simulink model "Design_5new_4weeks_Q3"  (R2026a)
settings: Solver=FixedStepAuto  StopTime=2419200  FixedStep=300
undefined symbols (not defined in the file): coloring, m, n, tamk, vapor
libraries: mqttlib x7
(part 1 of 2)
settings Model: Creator=User  LastModifiedBy=User
settings ConfigComp: PLC_TargetIDE=codesys35  PLC_MultiTBSigbuilderTimeRange=off  PLC_FoldFBCallOutputVar=off  PLC_RemoveUnusedSSMethodCallArguments=off  PLC_UseCallOutputArgSyntax=off  PLC_EnableUnsignedAndDoubleTypes=off  PLC_EnableUDTSplitting=off  PLC_MaxFieldsInUDT=500.0  PLC_InlineEnumCastFunction=off  PLC_RTWMaxIdLength=31.0  PLC_RollThreshold=5.0  PLC_ActiveTab=0.0  PLC_EnableStringLiteralTB=on  PLC_Enable64bitIntSupport=off

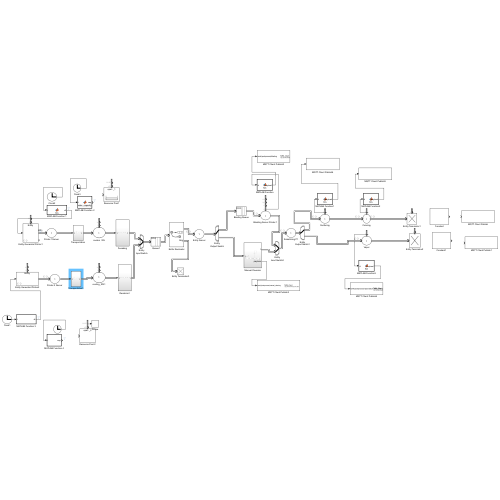
[thumbnail: Simulink's stored preview of the top-level diagram]
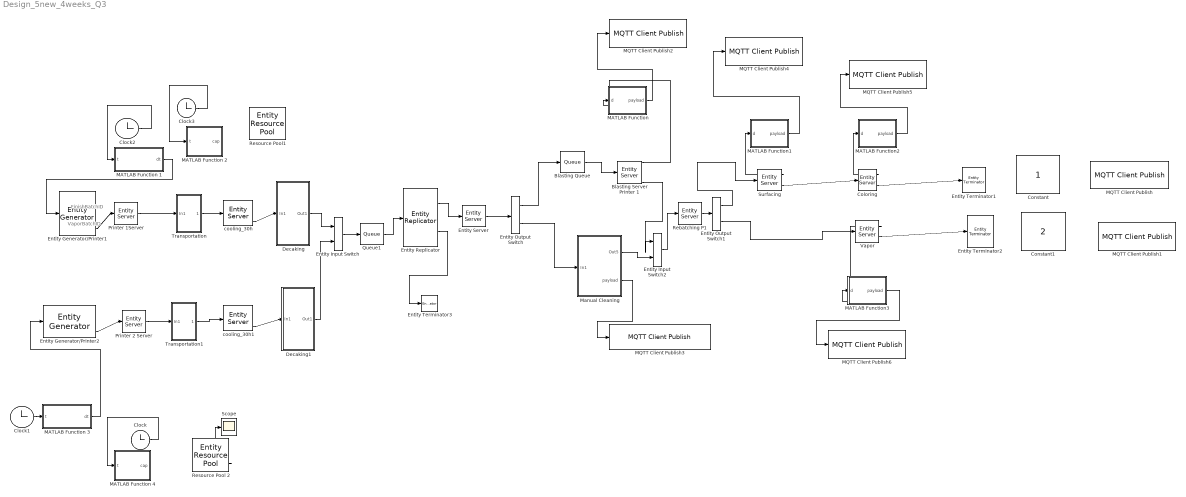
== system Design_5new_4weeks_Q3 ==
  note: VaporBatchID
  note: FinishBatchID
  " Queue1" : Queue  InputPortMessageModes=m  OutputPortMessageModes=m
  Blasting Queue : Queue  InputPortMessageModes=m  OutputPortMessageModes=m
  Blasting Server Printer 1 : EntityServer  InputPortMessageModes=m  OutputPortMessageModes=n,n,n,n,m  Capacity=1  ServiceTimeValue=8*60  EntryAction=|  NumberEntitiesDeparted=on  NumberEntitiesInBlock=on  NumberEntitiesPending=on  NumEntitiesExtracted=on
      | % =========================================================
      | % BLASTING PROCESS : PowerShot C
      | % Supervisor Excel Values
      | % Simulink-safe version
      | % =========================================================
      | 
      | entity.prev_proc = 3;          % 3 = Blasting completed
      | 
      | % Supervisor values
      | entity.operator_time_min = 1;  % min/batch
      | entity.capacity_L = 5;         % L/batch
      | entity.process_time_min = 8;   % min
      | entity.power = 5;              % kW
      | 
      | % Energy calculation
      | entity.energy = ...
      |     entity.power * entity.process_time_min / 60;
      | 
      | % Accumulate totals
      | entity.total_energy = ...
      |     entity.total_energy + entity.energy;
      | 
      | entity.total_operator_min = ...
      |     entity.total_operator_min + entity.operator_time_min;
      | 
      | % Debug print
      | fprintf(['[BLASTING CHECK] ' ...
      |     'SourceID=%g | BuildID=%g | BatchID=%g | PartID=%g | ' ...
      |     'PrevProc=%g | Volume=%.2f | Capacity=%.2f | ' ...
      |     'ProcessTime=%.2f min | Operator=%.2f min | ' ...
      |     'Power=%.2f kW | Energy=%.3f kWh | ' ...
      |     'TotalEnergy=%.3f kWh | TotalOperator=%.3f min\n'], ...
      |     entity.SourceID, ...
      |     entity.BuildID, ...
      |     entity.BatchID, ...
      |     entity.PartID, ...
      |     entity.prev_proc, ...
      |     entity.part_volume, ...
      |     entity.capacity_L, ...
      |     entity.process_time_min, ...
      |     entity.operator_time_min, ...
      |     entity.power, ...
      |     entity.energy, ...
      |     entity.total_energy, ...
      |     entity.total_operator_min);
      settings: OutputPortMap=o0,o1,o3,o12,o9
  Clock{,1..3} (4 alike) : Clock
  Coloring : EntityServer  InputPortMessageModes=m  OutputPortMessageModes=n,m  Capacity=1  ServiceTimeValue=150*60  EntryAction=|  ExitAction=|  NumberEntitiesDeparted=on
      EntryAction=|
      | %#codegen
      | 
      | % =========================================================
      | % SURFACING PROCESS : PowerShot S
      | % Supervisor Excel Values
      | % Simulink-safe version
      | % =========================================================
      | 
      | persistent surfacingBatchCounter
      | 
      | if isempty(surfacingBatchCounter)
      |     surfacingBatchCounter = 9000;    % first SurfacingBatchID = 9001
      | end
      | 
      | % =========================================================
      | % DUPLICATE PROTECTION
      | % If this entity already completed Surfacing, do not add energy again
      | % =========================================================
      | if entity.prev_proc == 5
      | 
      |     fprintf(['[SURFACING SKIPPED - ALREADY DONE] ' ...
      |         'SourceID=%g | BuildID=%g | PartID=%g | BatchID=%g | TotalEnergy=%.3f\n'], ...
      |         entity.SourceID, ...
      |         entity.BuildID, ...
      |         entity.PartID, ...
      |         entity.BatchID, ...
      |         entity.total_energy);
      | 
      | else
      | 
      |     % =====================================================
      |     % PROCESS IDENTIFICATION
      |     % =====================================================
      |     entity.prev_proc = 5;          % 5 = Surfacing completed
      |     entity.process_name = 5;
      | 
      |     % =====================================================
      |     % SUPERVISOR VALUES
      |     % =====================================================
      |     entity.operator_time_min = 1;  % min/batch
      |     entity.capacity_L = 5;         % L/batch
      |     entity.process_time_min = 10;  % min
      |     entity.power = 5;              % kW
      | 
      |     % =====================================================
      |     % ENERGY CALCULATION
      |     % =====================================================
      |     entity.energy = entity.power * entity.process_time_min / 60;
      | 
      |     % =====================================================
      |     % ACCUMULATE TOTALS
      |     % =====================================================
      |     entity.total_energy = entity.total_energy + entity.energy;
      | 
      |     entity.total_operator_min = ...
      |         entity.total_operator_min + entity.operator_time_min;
      | 
      |     % =====================================================
      |     % NEW BATCH ID AFTER SURFACING
      |     % Coloring receives this BatchID
      |     % =====================================================
      |     surfacingBatchCounter = surfacingBatchCounter + 1;
      | 
      |     entity.surfacing_batch_id = surfacingBatchCounter;
      |     entity.SurfaceBatchID = surfacingBatchCounter;
      | 
      |     % Current active BatchID after Surfacing
      |     entity.BatchID = entity.surfacing_batch_id;
      | 
      |     % Keep route marker for Coloring path
      |     entity.finish_type = 1;
      | 
      |     % =====================================================
      |     % DEBUG PRINT
      |     % =====================================================
      |     fprintf(['[SURFACING CHECK] ' ...
      |         'SourceID=%g | BuildID=%g | BatchID=%g | ' ...
      |         'SurfacingBatchID=%g | ColoringInputBatchID=%g | ' ...
      |         'PartID=%g | PrevProc=%g | FinishType=%g | Volume=%.2f | Capacity=%.2f | ' ...
      |         'ProcessTime=%.2f min | Operator=%.2f min | ' ...
      |         'Power=%.2f kW | Energy=%.3f kWh | ' ...
      |         'TotalEnergy=%.3f kWh | TotalOperator=%.3f min\n'], ...
      |         entity.SourceID, ...
      |         entity.BuildID, ...
      |         entity.BatchID, ...
      |         entity.surfacing_batch_id, ...
      |         entity.BatchID, ...
      |         entity.PartID, ...
      |         entity.prev_proc, ...
      |         entity.finish_type, ...
      |         entity.part_volume, ...
      |         entity.capacity_L, ...
      |         entity.process_time_min, ...
      |         entity.operator_time_min, ...
      |         entity.power, ...
      |         entity.energy, ...
      |         entity.total_energy, ...
      |         entity.total_operator_min);
      | 
      | end
      ExitAction=|
      | fprintf('[COLORING CHECK] PartID=%g | BatchID=%g\n', ...
      |     entity.PartID, ...
      |     entity.BatchID);
      settings: OutputPortMap=o0,o9
  Constant : Constant  SampleTime=300
  Constant1 : Constant  Value=2  SampleTime=300
  Decaking : Subsystem
  Decaking1 : Subsystem
  Entity Input Switch : EntityInputSwitch  InputPortMessageModes=m,m  OutputPortMessageModes=m
  Entity Input Switch2 : EntityInputSwitch  InputPortMessageModes=m,m  OutputPortMessageModes=m
  Entity Output Switch : EntityOutputSwitch  InputPortMessageModes=m  OutputPortMessageModes=m,m  SwitchingCriterion=From attribute  SwitchAttributeName=route_dp
  Entity Output Switch1 : EntityOutputSwitch  InputPortMessageModes=m  OutputPortMessageModes=m,m  SwitchingCriterion=From attribute  SwitchAttributeName=finish_type
  Entity Generator/Printer1 : EntityGenerator  OutputPortMessageModes=n,n,m  TimeSource=Signal port  GenerateAction=|  AttributeName=BatchID|PartID|material_type|finish_type|prev_proc|SourceID|route_dp|BuildID|part_volume|blast_batch_id|manual_batch_id|surface_batch_id|vapor_batch_id|Build_Time|Build_Volume|Build_schedule|Primary_powder|Secondary_powder|Inert_gas_cons|Electricity_cons|Comp_air_cons|Fill_ratio|Build_height|Laser_power|Total_print_mass|Heat_loss|process_time_min|operator_time_min|capacity_L|power|energy|transport_time_min|total_energy|total_operator_min|process_name|energy_stage|finish_batch_id|PrinterBatchID|DecakingBatchID|RouteID|FinishBatchI|ColorBatchID|FinalBatchID|BlastBatchID|ManualBatchID|FinishBatchID|SurfaceBatchID|VaporBatchID|printer_batch_id|color_batch_id|surfacing_batch_id  AttributeInitialValue=0|0|1|2|1|0|1|0|0|0|0|0|0|0|0|1|0|0|0|0|0|0|0|0|0|0|0|0|0|0|0|10|0|0|0|0|0|0|0|0|0|0|0|0|0|0|0|0|0|0|0  NumberEntitiesDeparted=on  AverageIntergenerationTime=on  EntityType=Structured  EntityTypeName=Entity
      | %#codegen
      | 
      | persistent batchCounter1 printer1PrintDone
      | 
      | % =========================================================
      | % INIT
      | % =========================================================
      | if isempty(batchCounter1)
      |     batchCounter1 = 0;
      | end
      | 
      | if isempty(printer1PrintDone)
      |     printer1PrintDone = false;
      | end
      | 
      | batchCounter1 = batchCounter1 + 1;
      | 
      | % =========================================================
      | % BASIC IDs
      | % =========================================================
      | entity.SourceID = 1;
      | entity.PartID   = 0;
      | 
      | entity.BuildID = batchCounter1;
      | entity.BatchID = 0;
      | 
      | % =========================================================
      | % INITIALIZE ALL BATCH FIELDS
      | % =========================================================
      | entity.PrinterBatchID  = batchCounter1;
      | entity.DecakingBatchID = 0;
      | entity.RouteID         = 0;
      | 
      | entity.BlastBatchID    = 0;
      | entity.ManualBatchID   = 0;
      | entity.FinishBatchID   = 0;
      | entity.SurfaceBatchID  = 0;
      | entity.VaporBatchID    = 0;
      | entity.ColorBatchID    = 0;
      | entity.FinalBatchID    = 0;
      | 
      | % lowercase fields, if used in later blocks
      | entity.printer_batch_id   = batchCounter1;
      | entity.color_batch_id     = 0;
      | entity.surfacing_batch_id = 0;
      | 
      | % =========================================================
      | % BUILD / PRINTER
      | % =========================================================
      | entity.Build_Time     = 1200;      % min = 20 h
      | entity.Build_Volume   = 10000;     % cm3
      | entity.Build_schedule = 1;
      | 
      | % =========================================================
      | % PART
      | % =========================================================
      | entity.part_volume   = 0;
      | entity.material_type = 1;
      | 
      | % =========================================================
      | % ROUTING DEFAULTS
      | % =========================================================
      | entity.prev_proc   = 1;    % 1 = Printing completed
      | entity.route_dp    = 1;
      | entity.finish_type = 1;
      | 
      | % =========================================================
      | % PROCESS PARAMETERS
      | % =========================================================
      | entity.power            = 2;       % kW
      | entity.process_time_min = 1200;    % min
      | 
      | % =========================================================
      | % ENERGY
      | % =========================================================
      | entity.energy = entity.power * entity.process_time_min / 60;
      | entity.total_energy = entity.energy;
      | 
      | % =========================================================
      | % OPERATOR / TRANSPORT
      | % =========================================================
      | entity.operator_time_min  = 0;
      | entity.capacity_L         = 0;
      | entity.transport_time_min = 10;
      | entity.total_operator_min = 0;
      | 
      | % =========================================================
      | % DEBUG / TRACKING
      | % =========================================================
      | entity.energy_stage = 1;
      | entity.process_name = 1;
      | 
      | % =========================================================
      | % DEBUG PRINT ONLY ONCE
      | % =========================================================
      | if ~printer1PrintDone
      |     fprintf('[Printer1 INIT] SourceID=%g | BuildID=%g | BatchID=%g | PrinterBatchID=%g | PartID=%g | BuildTime=%g min | Energy=%.3f | Total=%.3f\n', ...
      |         entity.SourceID, ...
      |         entity.BuildID, ...
      |         entity.BatchID, ...
      |         entity.PrinterBatchID, ...
      |         entity.PartID, ...
      |         entity.process_time_min, ...
      |         entity.energy, ...
      |         entity.total_energy);
      | 
      |     printer1PrintDone = true;
      | end
      settings: InputPortMap=u1  OutputPortMap=o0,o2,o3
  Entity Generator/Printer2 : EntityGenerator  OutputPortMessageModes=n,n,m  TimeSource=Signal port  GenerateAction=|  AttributeName=BatchID|PartID|material_type|finish_type|prev_proc|SourceID|route_dp|BuildID|part_volume|blast_batch_id|manual_batch_id|surface_batch_id|vapor_batch_id|Build_Time|Build_Volume|Build_schedule|Primary_powder|Secondary_powder|Inert_gas_cons|Electricity_cons|Comp_air_cons|Fill_ratio|Build_height|Laser_power|Total_print_mass|Heat_loss|process_time_min|operator_time_min|capacity_L|power|energy|transport_time_min|total_energy|total_operator_min|process_name|energy_stage|finish_batch_id|PrinterBatchID|DecakingBatchID|RouteID|FinishBatchI|ColorBatchID|FinalBatchID|BlastBatchID|ManualBatchID|FinishBatchID|SurfaceBatchID|VaporBatchID|printer_batch_id|color_batch_id|surfacing_batch_id  AttributeInitialValue=0|1|0|2|1|0|1|0|0|0|0|0|0|0|0|1|0|0|0|0|0|0|0|0|0|0|0|0|0|0|0|10|0|0|0|0|0|0|0|0|0|0|0|0|0|0|0|0|0|0|0  NumberEntitiesDeparted=on  AverageIntergenerationTime=on  EntityType=Structured  EntityTypeName=Entity
      | %#codegen
      | 
      | persistent batchCounter2 printer2PrintDone
      | 
      | % =========================================================
      | % INIT
      | % =========================================================
      | if isempty(batchCounter2)
      |     batchCounter2 = 999;      % first BuildID = 1000
      | end
      | 
      | if isempty(printer2PrintDone)
      |     printer2PrintDone = false;
      | end
      | 
      | batchCounter2 = batchCounter2 + 1;
      | 
      | % =========================================================
      | % BASIC IDs
      | % =========================================================
      | entity.SourceID = 2;
      | entity.PartID   = 0;
      | 
      | % Build tracking
      | entity.BuildID = batchCounter2;
      | 
      | % Current/latest batch ID
      | entity.BatchID = 0;
      | 
      | % =========================================================
      | % INITIALIZE ALL BATCH FIELDS
      | % =========================================================
      | entity.PrinterBatchID  = batchCounter2;
      | entity.DecakingBatchID = 0;
      | entity.RouteID         = 0;
      | 
      | entity.BlastBatchID    = 0;
      | entity.ManualBatchID   = 0;
      | 
      | entity.FinishBatchID   = 0;
      | entity.SurfaceBatchID  = 0;
      | entity.VaporBatchID    = 0;
      | 
      | entity.ColorBatchID    = 0;
      | entity.FinalBatchID    = 0;
      | 
      | % lowercase versions used later in model
      | entity.printer_batch_id   = batchCounter2;
      | entity.color_batch_id     = 0;
      | entity.surfacing_batch_id = 0;
      | 
      | % =========================================================
      | % PRINTER / BUILD
      | % =========================================================
      | entity.Build_Time     = 1440;      % min = 24 h
      | entity.Build_Volume   = 10000;     % cm3
      | entity.Build_schedule = 1;
      | 
      | % =========================================================
      | % PART - ASSIGNED LATER
      | % =========================================================
      | entity.part_volume   = 0;
      | entity.material_type = 1;
      | 
      | % =========================================================
      | % MATERIAL / CONSUMPTION - INITIAL VALUES
      | % =========================================================
      | entity.Primary_powder   = 0;
      | entity.Secondary_powder = 0;
      | 
      | entity.Inert_gas_cons   = 0;
      | entity.Electricity_cons = 0;
      | entity.Comp_air_cons    = 0;
      | 
      | entity.Fill_ratio       = 0;
      | entity.Build_height     = 0;
      | 
      | entity.Laser_power      = 0;
      | entity.Total_print_mass = 0;
      | entity.Heat_loss        = 0;
      | 
      | % =========================================================
      | % ROUTING DEFAULT VALUES
      | % =========================================================
      | entity.prev_proc   = 1;      % 1 = Printing completed
      | entity.route_dp    = 1;
      | entity.finish_type = 1;
      | 
      | % =========================================================
      | % ENERGY
      | % =========================================================
      | entity.power = 2;                 % kW
      | 
      | entity.process_time_min = 1440;   % min
      | 
      | % Printer energy calculation
      | entity.energy = ...
      |     entity.power * entity.process_time_min / 60;
      | 
      | % Initialize total energy
      | entity.total_energy = entity.energy;
      | 
      | % =========================================================
      | % OTHER PROCESS ATTRIBUTES
      | % =========================================================
      | entity.operator_time_min  = 0;
      | 
      | entity.capacity_L         = 0;
      | 
      | entity.transport_time_min = 10;
      | 
      | entity.total_operator_min = 0;
      | 
      | % =========================================================
      | % DEBUG / TRACKING
      | % =========================================================
      | entity.energy_stage = 1;
      | 
      | entity.process_name = 1;
      | 
      | % =========================================================
      | % DEBUG PRINT ONLY ONE TIME
      | % =========================================================
      | if ~printer2PrintDone
      | 
      |     fprintf('[Printer2 INIT] SourceID=%g | BuildID=%g | BatchID=%g | PrinterBatchID=%g | PartID=%g | BuildTime=%g min | Energy=%.3f | Total=%.3f\n', ...
      |         entity.SourceID, ...
      |         entity.BuildID, ...
      |         entity.BatchID, ...
      |         entity.PrinterBatchID, ...
      |         entity.PartID, ...
      |         entity.process_time_min, ...
      |         entity.energy, ...
      |         entity.total_energy);
      | 
      |     printer2PrintDone = true;
      | 
      | end
      settings: InputPortMap=u1  OutputPortMap=o0,o2,o3
  Entity Replicator : EntityReplicator  InputPortMessageModes=m  OutputPortMessageModes=m,m  ReplicasDepartFrom=Single output port  NumberReplicas=5  HoldOriginalEntityUntilAllReplicasDepart=on
  Entity Server : EntityServer  InputPortMessageModes=m  OutputPortMessageModes=m  Capacity=1  EntryAction=|
      | persistent partCounterP1 partCounterP2
      | persistent blastBatchCounter manualBatchCounter
      | 
      | % =========================================================
      | % INIT
      | % =========================================================
      | if isempty(partCounterP1)
      |     partCounterP1 = 0;
      | end
      | 
      | if isempty(partCounterP2)
      |     partCounterP2 = 0;
      | end
      | 
      | % =========================================================
      | % NEW BATCH COUNTERS
      | % =========================================================
      | if isempty(blastBatchCounter)
      |     blastBatchCounter = 3000;
      | end
      | 
      | if isempty(manualBatchCounter)
      |     manualBatchCounter = 4000;
      | end
      | 
      | % =========================================================
      | % PART ASSIGNMENT AFTER REPLICATOR / MERGED LINE
      | % =========================================================
      | if entity.SourceID == 1
      | 
      |     partCounterP1 = partCounterP1 + 1;
      |     localIndex = mod(partCounterP1 - 1, 5) + 1;
      | 
      |     entity.PartID = localIndex;
      |     volume_map = [5 6 7 8 9];
      | 
      |     % Original printer batch
      |     entity.printer_batch_id = localIndex;
      | 
      | else
      | 
      |     partCounterP2 = partCounterP2 + 1;
      |     localIndex = mod(partCounterP2 - 1, 5) + 1;
      | 
      |     entity.PartID = localIndex + 5;
      |     volume_map = [10 11 12 13 14];
      | 
      |     % Original printer batch
      |     entity.printer_batch_id = 1000 + localIndex;
      | 
      | end
      | 
      | % =========================================================
      | % PART VOLUME
      | % =========================================================
      | entity.part_volume = volume_map(localIndex);
      | 
      | % =========================================================
      | % ROUTING LOGIC
      | % =========================================================
      | if localIndex <= 4
      | 
      |     % ============================================
      |     % BLASTING ROUTE
      |     % ============================================
      |     entity.route_dp = 1;
      |     entity.prev_proc = 1;
      | 
      |     % NEW blasting batch
      |     blastBatchCounter = blastBatchCounter + 1;
      | 
      |     entity.blast_batch_id = blastBatchCounter;
      |     entity.manual_batch_id = 0;
      | 
      |     % CURRENT ACTIVE BATCH
      |     entity.BatchID = entity.blast_batch_id;
      | 
      |     entity.process_name = 1;
      | 
      | else
      | 
      |     % ============================================
      |     % MANUAL CLEANING ROUTE
      |     % ============================================
      |     entity.route_dp = 2;
      |     entity.prev_proc = 2;
      | 
      |     % NEW manual cleaning batch
      |     manualBatchCounter = manualBatchCounter + 1;
      | 
      |     entity.manual_batch_id = manualBatchCounter;
      |     entity.blast_batch_id = 0;
      | 
      |     % CURRENT ACTIVE BATCH
      |     entity.BatchID = entity.manual_batch_id;
      | 
      |     entity.process_name = 2;
      | 
      | end
      | 
      | % =========================================================
      | % DEBUG PRINT
      | % =========================================================
      | fprintf(['[ASSIGN COMMON] SourceID=%g | BuildID=%g | ' ...
      |     'PrinterBatchID=%g | BatchID=%g | BlastBatchID=%g | ' ...
      |     'ManualBatchID=%g | PartID=%g | Volume=%.2f | ' ...
      |     'route_dp=%g | prev_proc=%g | process_name=%g | ' ...
      |     'total_energy=%.3f\n'], ...
      |     entity.SourceID, ...
      |     entity.BuildID, ...
      |     entity.printer_batch_id, ...
      |     entity.BatchID, ...
      |     entity.blast_batch_id, ...
      |     entity.manual_batch_id, ...
      |     entity.PartID, ...
      |     entity.part_volume, ...
      |     entity.route_dp, ...
      |     entity.prev_proc, ...
      |     entity.process_name, ...
      |     entity.total_energy);
  Entity Terminator1 : EntityTerminator  InputPortMessageModes=m  NumberEntitiesArrived=on
      settings: OutputPortMap=o0
  Entity Terminator2 : EntityTerminator  InputPortMessageModes=m  NumberEntitiesArrived=on
      settings: OutputPortMap=o0
  Entity Terminator3 : EntityTerminator  InputPortMessageModes=m
  MATLAB Function : MATLAB Function  TreatAsAtomicUnit=on
  MATLAB Function 1 : MATLAB Function  TreatAsAtomicUnit=on
  MATLAB Function 2 : MATLAB Function  TreatAsAtomicUnit=on
  MATLAB Function 3 : MATLAB Function  TreatAsAtomicUnit=on
  MATLAB Function 4 : MATLAB Function  TreatAsAtomicUnit=on
  MATLAB Function1 : MATLAB Function  TreatAsAtomicUnit=on
  MATLAB Function2 : MATLAB Function  TreatAsAtomicUnit=on
  MATLAB Function3 : MATLAB Function  TreatAsAtomicUnit=on
  MQTT Client Publish : mqttlib/MQTT Client Publish  RetainClient=TAMK_Client  ClientList=TAMK_Client  TopicsTable={ '1', 'tamk/coloring', '0', 'off' }  PublishOnDataChange=off  SampleTime=-1  TopicNames=tamk/coloring  NumTopics=1  IsLib=0  BlkName=MQTT Client Publish
  MQTT Client Publish1 : mqttlib/MQTT Client Publish  RetainClient=TAMK_Client  ClientList=TAMK_Client  TopicsTable={ '1', 'tamk/vapor', '0', 'off' }  PublishOnDataChange=off  SampleTime=-1  TopicNames=tamk/vapor  NumTopics=1  IsLib=0  BlkName=MQTT Client Publish
  MQTT Client Publish2 : mqttlib/MQTT Client Publish  RetainClient=TAMK_Client  ClientList=TAMK_Client  TopicsTable={ '1', 'tamk/postprocess/blasting', '0', 'off' }  PublishOnDataChange=on  SampleTime=-1  TopicNames=tamk/postprocess/blasting  NumTopics=1  IsLib=0  BlkName=MQTT Client Publish
  MQTT Client Publish3 : mqttlib/MQTT Client Publish  RetainClient=TAMK_Client  ClientList=TAMK_Client  TopicsTable={ '1', 'tamk/postprocess/manual_cleaning', '0', 'off' }  PublishOnDataChange=on  SampleTime=-1  TopicNames=tamk/postprocess/manual_cleaning  NumTopics=1  IsLib=0  BlkName=MQTT Client Publish
  MQTT Client Publish4 : mqttlib/MQTT Client Publish  RetainClient=TAMK_Client  ClientList=TAMK_Client  TopicsTable={ '1', 'tamk/postprocess/surfacing', '0', 'off' }  PublishOnDataChange=on  SampleTime=-1  TopicNames=tamk/postprocess/surfacing  NumTopics=1  IsLib=0  BlkName=MQTT Client Publish
  MQTT Client Publish5 : mqttlib/MQTT Client Publish  RetainClient=TAMK_Client  ClientList=TAMK_Client  TopicsTable={ '1', 'tamk/postprocess/coloring', '0', 'off' }  PublishOnDataChange=on  SampleTime=-1  TopicNames=tamk/postprocess/coloring  NumTopics=1  IsLib=0  BlkName=MQTT Client Publish
  MQTT Client Publish6 : mqttlib/MQTT Client Publish  RetainClient=TAMK_Client  ClientList=TAMK_Client  TopicsTable={ '1', 'tamk/postprocess/vapor/batch_10/source_2/build_1000/part_10/time_168/energy_42/total_90', '0', 'off' }  PublishOnDataChange=on  SampleTime=-1  TopicNames=tamk/postprocess/vapor/batch_10/source_2/build_1000/part_10/time_168/energy_42/total_90  NumTopics=1  IsLib=0  BlkName=MQTT Client Publish
  Manual Cleaning : Subsystem
  Printer 1Server : EntityServer  InputPortMessageModes=m  OutputPortMessageModes=m  Capacity=1  ServiceTimeValue=20*60*60  EntryAction=|
      | % Printer 1 Server
      | % Only service/time block. Do not add printer energy again.
      | 
      | entity.Build_Time = 20 * 60;   % minutes
      | 
      | % Keep existing energy from Entity Generator
      | % Do NOT use:
      | % entity.total_energy = entity.total_energy + entity.energy;
      | 
      | fprintf('[Printer1 Server] SourceID=%.0f | BuildID=%.0f | BatchID=%.0f | BuildTime=%.0f min | Energy=%.3f | Total=%.3f\n', ...
      |     entity.SourceID, ...
      |     entity.BuildID, ...
      |     entity.BatchID, ...
      |     entity.Build_Time, ...
      |     entity.energy, ...
      |     entity.total_energy);
  Printer 2 Server : EntityServer  InputPortMessageModes=m  OutputPortMessageModes=m  Capacity=1  ServiceTimeValue=24*60*60  EntryAction=|
      | % Printer 2 Server
      | % Only service/time block. Do not add printer energy again.
      | 
      | entity.Build_Time = 24 * 60;   % minutes
      | 
      | % Keep existing energy from Entity Generator
      | % Do NOT use:
      | % entity.total_energy = entity.total_energy + entity.energy;
      | 
      | fprintf('[Printer2 Server] SourceID=%.0f | BuildID=%.0f | BatchID=%.0f | BuildTime=%.0f min | Energy=%.3f | Total=%.3f\n', ...
      |     entity.SourceID, ...
      |     entity.BuildID, ...
      |     entity.BatchID, ...
      |     entity.Build_Time, ...
      |     entity.energy, ...
      |     entity.total_energy);
  Rebatching P1 : EntityServer  InputPortMessageModes=m  OutputPortMessageModes=m  Capacity=1  EntryAction=|
      | persistent finishBatchCounter finishRouteCounter
      | 
      | % =========================================================
      | % INIT
      | % =========================================================
      | if isempty(finishBatchCounter)
      |     finishBatchCounter = 6000;   % Finish routing batch starts from 6001
      | end
      | 
      | if isempty(finishRouteCounter)
      |     finishRouteCounter = 0;
      | end
      | 
      | % =========================================================
      | % NEW BATCH ID AFTER BLASTING + MANUAL CLEANING COMBINE
      | % =========================================================
      | finishBatchCounter = finishBatchCounter + 1;
      | 
      | entity.finish_batch_id = finishBatchCounter;
      | entity.BatchID = entity.finish_batch_id;   % current/latest batch id
      | 
      | % =========================================================
      | % CYCLIC ROUTING COUNTER
      | % 8/10 -> Surfacing + Coloring
      | % 2/10 -> Vapor
      | % =========================================================
      | finishRouteCounter = mod(finishRouteCounter,10) + 1;
      | 
      | if finishRouteCounter <= 8
      | 
      |     entity.finish_type = 1;      % Surfacing + Coloring
      | 
      | else
      | 
      |     entity.finish_type = 2;      % Vapor
      | 
      | end
      | 
      | % =========================================================
      | % DEBUG PRINT
      | % =========================================================
      | fprintf('[Finish Routing] SourceID=%g | BuildID=%g | NewBatchID=%g | FinishBatchID=%g | PartID=%g | finish_type=%g | TotalEnergy=%.3f\n', ...
      |     entity.SourceID, ...
      |     entity.BuildID, ...
      |     entity.BatchID, ...
      |     entity.finish_batch_id, ...
      |     entity.PartID, ...
      |     entity.finish_type, ...
      |     entity.total_energy);
  Resource Pool 2 : EntityResourcePool  InputPortMessageModes=m  ResourceName=operator_pool_2  ResourceAmountSource=Change amount through control port  InitialResourceAmount=1  AverageUtilization=on  AmountAvailable=on
      settings: OutputPortMap=o1,o2
  Resource Pool1 : EntityResourcePool  InputPortMessageModes=m  ResourceName=operator_pool_1  ResourceAmountSource=Change amount through control port  InitialResourceAmount=1  AverageUtilization=on  AmountAvailable=on
      settings: OutputPortMap=o1,o2
  Scope : Scope
      settings: ActiveDisplayYMinimum=0.5314818623241806  ActiveDisplayYMaximum=0.531629835020397
  Surfacing : EntityServer  InputPortMessageModes=m  OutputPortMessageModes=n,m  Capacity=1  ServiceTimeValue=10*60  EntryAction=|  NumberEntitiesDeparted=on
      | %#codegen
      | 
      | persistent surfacingBatchCounter
      | 
      | if isempty(surfacingBatchCounter)
      |     surfacingBatchCounter = 9000;
      | end
      | 
      | % =========================================================
      | % SURFACING COMPLETED
      | % =========================================================
      | entity.prev_proc = 5;          % 5 = Surfacing completed
      | entity.process_name = 5;
      | 
      | % =========================================================
      | % SUPERVISOR VALUES
      | % =========================================================
      | entity.operator_time_min = 1;
      | entity.capacity_L = 5;
      | entity.process_time_min = 10;
      | entity.power = 5;
      | 
      | % =========================================================
      | % ENERGY
      | % =========================================================
      | entity.energy = entity.power * entity.process_time_min / 60;
      | 
      | entity.total_energy = entity.total_energy + entity.energy;
      | 
      | entity.total_operator_min = ...
      |     entity.total_operator_min + entity.operator_time_min;
      | 
      | % =========================================================
      | % BATCH ID FOR COLORING INPUT
      | % =========================================================
      | surfacingBatchCounter = surfacingBatchCounter + 1;
      | 
      | entity.surfacing_batch_id = surfacingBatchCounter;
      | entity.SurfaceBatchID = surfacingBatchCounter;
      | 
      | entity.BatchID = entity.surfacing_batch_id;
      | 
      | % Coloring route marker
      | entity.finish_type = 1;        % 1 = Surfacing + Coloring path
      | 
      | % =========================================================
      | % DEBUG PRINT
      | % =========================================================
      | fprintf(['[SURFACING CHECK] ' ...
      |     'SourceID=%g | BuildID=%g | BatchID=%g | ' ...
      |     'SurfacingBatchID=%g | ColoringInputBatchID=%g | ' ...
      |     'PartID=%g | PrevProc=%g | Volume=%.2f | Capacity=%.2f | ' ...
      |     'ProcessTime=%.2f min | Operator=%.2f min | ' ...
      |     'Power=%.2f kW | Energy=%.3f kWh | ' ...
      |     'TotalEnergy=%.3f kWh | TotalOperator=%.3f min\n'], ...
      |     entity.SourceID, ...
      |     entity.BuildID, ...
      |     entity.BatchID, ...
      |     entity.surfacing_batch_id, ...
      |     entity.BatchID, ...
      |     entity.PartID, ...
      |     entity.prev_proc, ...
      |     entity.part_volume, ...
      |     entity.capacity_L, ...
      |     entity.process_time_min, ...
      |     entity.operator_time_min, ...
      |     entity.power, ...
      |     entity.energy, ...
      |     entity.total_energy, ...
      |     entity.total_operator_min);
      settings: OutputPortMap=o0,o9
  Transportation : Subsystem
  Transportation1 : Subsystem
  Vapor : EntityServer  InputPortMessageModes=m  OutputPortMessageModes=n,m  Capacity=1  ServiceTimeValue=120*60  EntryAction=|  NumberEntitiesDeparted=on
      | % =========================================================
      | % VAPOR SMOOTHING PROCESS : Powerfuse S
      | % Supervisor Excel Values
      | % Simulink-safe version
      | % =========================================================
      | 
      | entity.prev_proc = 6;          % 6 = Vapor smoothing completed
      | 
      | % Supervisor values
      | entity.operator_time_min = 10; % min/batch
      | entity.capacity_L = 10;        % >10 L/batch
      | entity.process_time_min = 120; % min
      | entity.power = 15;             % kW
      | 
      | % Energy calculation
      | entity.energy = ...
      |     entity.power * entity.process_time_min / 60;
      | 
      | % Accumulate totals
      | entity.total_energy = ...
      |     entity.total_energy + entity.energy;
      | 
      | entity.total_operator_min = ...
      |     entity.total_operator_min + entity.operator_time_min;
      | 
      | % Debug print
      | fprintf(['[VAPOR CHECK] ' ...
      |     'SourceID=%g | BuildID=%g | BatchID=%g | ' ...
      |     'PartID=%g | PrevProc=%g | Volume=%.2f | ' ...
      |     'Capacity=%.2f | ProcessTime=%.2f min | ' ...
      |     'Operator=%.2f min | Power=%.2f kW | ' ...
      |     'Energy=%.3f kWh | TotalEnergy=%.3f kWh | ' ...
      |     'TotalOperator=%.3f min\n'], ...
      |     entity.SourceID, ...
      |     entity.BuildID, ...
      |     entity.BatchID, ...
      |     entity.PartID, ...
      |     entity.prev_proc, ...
      |     entity.part_volume, ...
      |     entity.capacity_L, ...
      |     entity.process_time_min, ...
      |     entity.operator_time_min, ...
      |     entity.power, ...
      |     entity.energy, ...
      |     entity.total_energy, ...
      |     entity.total_operator_min);
      | 
      | % Final output
      | fprintf(['[FINAL OUTPUT - VAPOR] ' ...
      |     'SourceID=%g | BuildID=%g | BatchID=%g | ' ...
      |     'PartID=%g | Volume=%.2f | ' ...
      |     'TotalEnergy=%.3f kWh | TotalOperator=%.3f min | ' ...
      |     'FinishType=%g\n'], ...
      |     entity.SourceID, ...
      |     entity.BuildID, ...
      |     entity.BatchID, ...
      |     entity.PartID, ...
      |     entity.part_volume, ...
      |     entity.total_energy, ...
      |     entity.total_operator_min, ...
      |     entity.finish_type);
      | 
      | % Process output
      | fprintf(['[PROCESS OUTPUT - VAPOR] ' ...
      |     'SourceID=%g | BuildID=%g | BatchID=%g | ' ...
      |     'PartID=%g | Volume=%.2f | Capacity=%.2f | ' ...
      |     'ProcessTime=%.2f min | OperatorTime=%.2f min | ' ...
      |     'Power=%.2f kW | Energy=%.3f kWh | ' ...
      |     'TotalEnergy=%.3f kWh\n'], ...
      |     entity.SourceID, ...
      |     entity.BuildID, ...
      |     entity.BatchID, ...
      |     entity.PartID, ...
      |     entity.part_volume, ...
      |     entity.capacity_L, ...
      |     entity.process_time_min, ...
      |     entity.operator_time_min, ...
      |     entity.power, ...
      |     entity.energy, ...
      |     entity.total_energy);
      settings: OutputPortMap=o0,o9
  cooling_30h : EntityServer  InputPortMessageModes=m  OutputPortMessageModes=n,n,m  Capacity=1  ServiceTimeValue=30*3600  NumberEntitiesInBlock=on  AverageWait=on
      settings: OutputPortMap=o1,o4,o9
  cooling_30h1 : EntityServer  InputPortMessageModes=m  OutputPortMessageModes=n,n,m  Capacity=1  ServiceTimeValue=30*3600  NumberEntitiesInBlock=on  AverageWait=on
      settings: OutputPortMap=o1,o4,o9
  wires:
  Clock/1 -> MATLAB Function 4/1(t)
  Clock1/1 -> MATLAB Function 3/1(t)
  MATLAB Function 3/1(dt) -> Entity Generator/Printer2/1
  cooling_30h/3 -> Decaking/1(In1)
  Resource Pool 2/2 -> Scope/1
  Entity Replicator/2 -> Entity Terminator3/1
  Coloring/2 -> Entity Terminator1/1
  Entity Output Switch1/2 -> Vapor/1
  Vapor/2 -> Entity Terminator2/1
  Surfacing/2 -> Coloring/1
  Entity Output Switch/2 -> Manual Cleaning/1(In1)
  Manual Cleaning/1(Out5) -> Entity Input Switch2/2
  Entity Generator/Printer1/3 -> Printer 1Server/1
  Entity Generator/Printer2/3 -> Printer 2 Server/1
  Blasting Queue/1 -> Blasting Server Printer 1/1
  Blasting Server Printer 1/5 -> Entity Input Switch2/1
  Entity Output Switch/1 -> Blasting Queue/1
  Transportation/1(Out1) -> cooling_30h/1
  Entity Server/1 -> Entity Output Switch/1
  Entity Input Switch2/1 -> Rebatching P1/1
  Printer 1Server/1 -> Transportation/1(In1)
  Clock2/1 -> MATLAB Function 1/1(t)
  Clock3/1 -> MATLAB Function 2/1(t)
  MATLAB Function 1/1(dt) -> Entity Generator/Printer1/1
  Printer 2 Server/1 -> Transportation1/1(In1)
  Transportation1/1(Out1) -> cooling_30h1/1
  cooling_30h1/3 -> Decaking1/1(In1)
  Rebatching P1/1 -> Entity Output Switch1/1
  Decaking1/1(Out1) -> Entity Input Switch/2
  Decaking/1(Out1) -> Entity Input Switch/1
  Entity Input Switch/1 -> " Queue1"/1
  " Queue1"/1 -> Entity Replicator/1
  Entity Replicator/1 -> Entity Server/1
  Blasting Server Printer 1/1 -> MATLAB Function/1(d)
  Surfacing/1 -> MATLAB Function1/1(d)
  Coloring/1 -> MATLAB Function2/1(d)
  Vapor/1 -> MATLAB Function3/1(d)
  MATLAB Function/1(payload) -> MQTT Client Publish2/1
  MATLAB Function1/1(payload) -> MQTT Client Publish4/1
  MATLAB Function2/1(payload) -> MQTT Client Publish5/1
  Manual Cleaning/2(payload) -> MQTT Client Publish3/1
  MATLAB Function3/1(payload) -> MQTT Client Publish6/1
  Entity Output Switch1/1 -> Surfacing/1

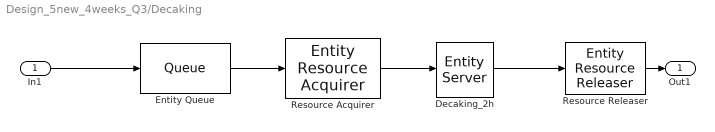
== system Design_5new_4weeks_Q3/Decaking ==
  In1 : Inport
  Decaking_2h : EntityServer  InputPortMessageModes=m  OutputPortMessageModes=m  Capacity=1  ServiceTimeValue=2*3600
  Entity Queue : Queue  InputPortMessageModes=m  OutputPortMessageModes=m
  Resource Acquirer : EntityResourceAcquirer  InputPortMessageModes=m  OutputPortMessageModes=m  ResourceName=operator_pool_1
      settings: OutputPortMap=o3
  Resource Releaser : EntityResourceReleaser  InputPortMessageModes=m  OutputPortMessageModes=m
  Out1 : Outport
  wires:
  In1/1 -> Entity Queue/1
  Entity Queue/1 -> Resource Acquirer/1
  Resource Acquirer/1 -> Decaking_2h/1
  Decaking_2h/1 -> Resource Releaser/1
  Resource Releaser/1 -> Out1/1

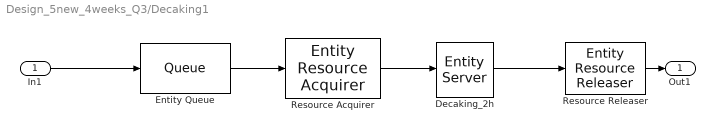
== system Design_5new_4weeks_Q3/Decaking1 ==
  In1 : Inport
  Decaking_2h : EntityServer  InputPortMessageModes=m  OutputPortMessageModes=m  Capacity=1  ServiceTimeValue=2*3600
  Entity Queue : Queue  InputPortMessageModes=m  OutputPortMessageModes=m
  Resource Acquirer : EntityResourceAcquirer  InputPortMessageModes=m  OutputPortMessageModes=m  ResourceName=operator_pool_2
      settings: OutputPortMap=o3
  Resource Releaser : EntityResourceReleaser  InputPortMessageModes=m  OutputPortMessageModes=m
  Out1 : Outport
  wires:
  In1/1 -> Entity Queue/1
  Entity Queue/1 -> Resource Acquirer/1
  Resource Acquirer/1 -> Decaking_2h/1
  Decaking_2h/1 -> Resource Releaser/1
  Resource Releaser/1 -> Out1/1

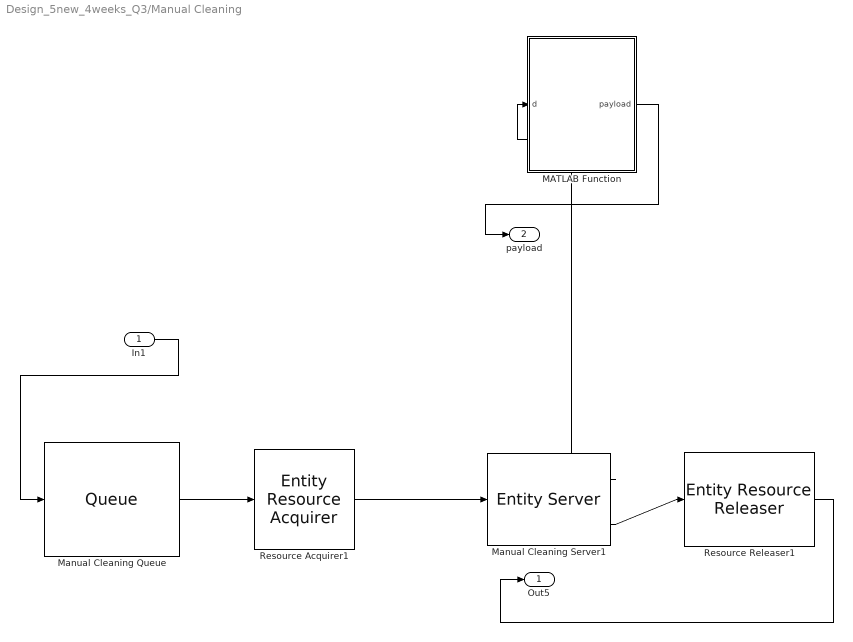
== system Design_5new_4weeks_Q3/Manual Cleaning ==
  In1 : Inport
  MATLAB Function : MATLAB Function  TreatAsAtomicUnit=on
  Manual Cleaning Queue : Queue  InputPortMessageModes=m  OutputPortMessageModes=m
  Manual Cleaning Server1 : EntityServer  InputPortMessageModes=m  OutputPortMessageModes=n,m  Capacity=1  ServiceTimeValue=30*60  EntryAction=|  NumberEntitiesDeparted=on
      | % =========================================================
      | % MANUAL CLEANING PROCESS
      | % Supervisor Excel Values
      | % Simulink-safe version
      | % =========================================================
      | 
      | entity.prev_proc = 4;          % 4 = Manual Cleaning completed
      | 
      | % Supervisor values
      | entity.operator_time_min = 30; % min/batch
      | entity.capacity_L = entity.part_volume;
      | entity.process_time_min = 30;  % min
      | entity.power = 0;              % kW
      | 
      | % Energy calculation
      | entity.energy = 0;
      | 
      | % Accumulate totals
      | entity.total_energy = ...
      |     entity.total_energy + entity.energy;
      | 
      | entity.total_operator_min = ...
      |     entity.total_operator_min + entity.operator_time_min;
      | 
      | % Debug print
      | fprintf(['[MANUAL CLEANING CHECK] ' ...
      |     'SourceID=%g | BuildID=%g | BatchID=%g | PartID=%g | ' ...
      |     'PrevProc=%g | Volume=%.2f | Capacity=%.2f | ' ...
      |     'ProcessTime=%.2f min | Operator=%.2f min | ' ...
      |     'Power=%.2f kW | Energy=%.3f kWh | ' ...
      |     'TotalEnergy=%.3f kWh | TotalOperator=%.3f min\n'], ...
      |     entity.SourceID, ...
      |     entity.BuildID, ...
      |     entity.BatchID, ...
      |     entity.PartID, ...
      |     entity.prev_proc, ...
      |     entity.part_volume, ...
      |     entity.capacity_L, ...
      |     entity.process_time_min, ...
      |     entity.operator_time_min, ...
      |     entity.power, ...
      |     entity.energy, ...
      |     entity.total_energy, ...
      |     entity.total_operator_min);
      settings: OutputPortMap=o0,o9
  Resource Acquirer1 : EntityResourceAcquirer  InputPortMessageModes=m  OutputPortMessageModes=m  ResourceName=operator_pool_1
      settings: OutputPortMap=o3
  Resource Releaser1 : EntityResourceReleaser  InputPortMessageModes=m  OutputPortMessageModes=m
  Out5 : Outport
  payload : Outport  Port=2
  wires:
  Manual Cleaning Server1/2 -> Resource Releaser1/1
  In1/1 -> Manual Cleaning Queue/1
  Resource Acquirer1/1 -> Manual Cleaning Server1/1
  Manual Cleaning Queue/1 -> Resource Acquirer1/1
  Resource Releaser1/1 -> Out5/1
  Manual Cleaning Server1/1 -> MATLAB Function/1(d)
  MATLAB Function/1(payload) -> payload/1

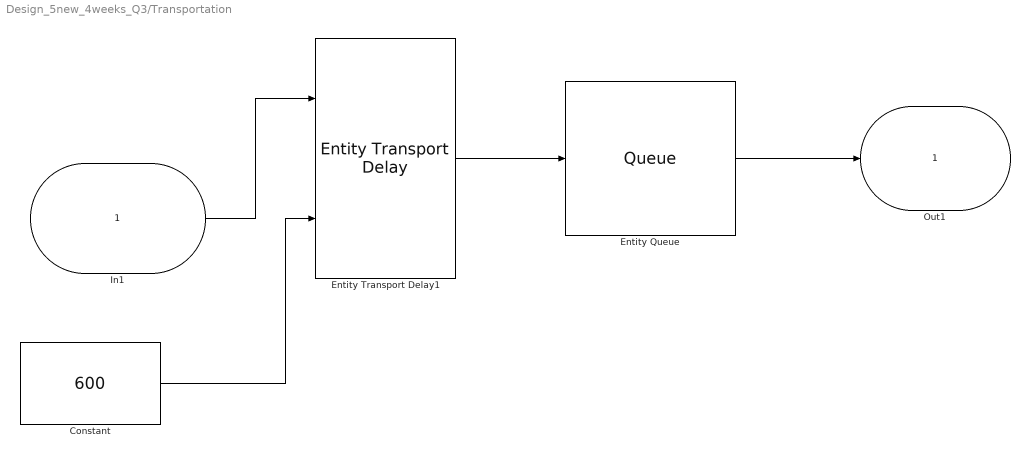
== system Design_5new_4weeks_Q3/Transportation ==
  In1 : Inport
  Constant : Constant  Value=600
  Entity Transport Delay1 : EntityTransportDelay  InputPortMessageModes=m,n  OutputPortMessageModes=m
  Entity Queue : Queue  InputPortMessageModes=m  OutputPortMessageModes=m
  Out1 : Outport
  wires:
  Entity Transport Delay1/1 -> Entity Queue/1
  In1/1 -> Entity Transport Delay1/1
  Constant/1 -> Entity Transport Delay1/2
  Entity Queue/1 -> Out1/1

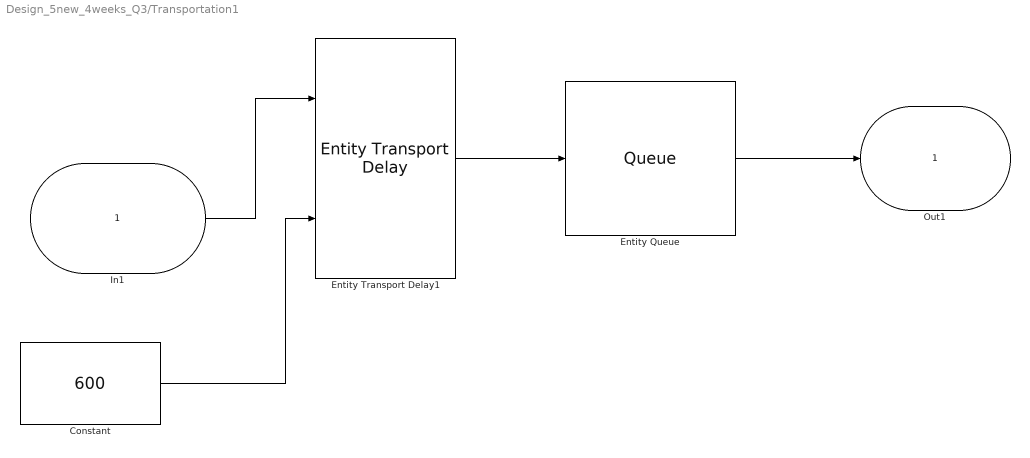
== system Design_5new_4weeks_Q3/Transportation1 ==
  In1 : Inport
  Constant : Constant  Value=600
  Entity Transport Delay1 : EntityTransportDelay  InputPortMessageModes=m,n  OutputPortMessageModes=m
  Entity Queue : Queue  InputPortMessageModes=m  OutputPortMessageModes=m
  Out1 : Outport
  wires:
  Entity Transport Delay1/1 -> Entity Queue/1
  In1/1 -> Entity Transport Delay1/1
  Constant/1 -> Entity Transport Delay1/2
  Entity Queue/1 -> Out1/1

== matlab function Design_5new_4weeks_Q3/MATLAB Function 3 ==
  data: t input; dt output



function dt = fcn_printer2(t)
%#codegen

SEC_PER_DAY = 24*3600;
rel_sec = 8*3600;    % Same as Printer 1 → 08:00 AM
epsT = 1e-9;

day  = floor(t/SEC_PER_DAY);
tod  = mod(t, SEC_PER_DAY);

next_day = day;

while true
    ndow  = mod(next_day,7);      % day of week
    nweek = floor(next_day/7);    % week index

    % Skip weekends
    if ndow == 5 || ndow == 6
        next_day = next_day + 1;
        continue;
    end

    % Skip first Monday of week 1
    if (nweek == 0) && (ndow == 0)
        next_day = next_day + 1;
        continue;
    end

    % Check today's time
    if next_day == day
        if tod < rel_sec - epsT
            break;   % release today at 08:00
        else
            next_day = next_day + 1;
            continue;
        end
    else
        break;
    end
end

next_release = next_day*SEC_PER_DAY + rel_sec;

% Ensure positive time step
dt = max(next_release - t, 1e-6);

end

== matlab function Design_5new_4weeks_Q3/MATLAB Function 4 ==
  data: t input; cap output




function cap = operator_capacity_p2(t)
%#codegen

SEC_PER_DAY = 24*3600;

day = floor(t/SEC_PER_DAY);     % Day index
tod = mod(t, SEC_PER_DAY);      % Time of day (seconds)
dow = mod(day,7);               % Day of week (0=Mon,...,6=Sun)
week = floor(day/7);            % Week index

% --- Weekend: no operator ---
if dow >= 5
    cap = 0;
    return;
end

% --- Special case: First Monday (week 0) ---
if (week == 0) && (dow == 0)
    % Only 12:00–16:00
    if tod >= 12*3600 && tod < 16*3600
        cap = 1;
    else
        cap = 0;
    end
else
    % Normal weekdays: 08:00–16:00
    if tod >= 8*3600 && tod < 16*3600
        cap = 1;
    else
        cap = 0;
    end
end

end

== matlab function Design_5new_4weeks_Q3/MATLAB Function 1 ==
  data: t input; dt output



function dt = fcn(t)
%#codegen

SEC_PER_DAY = 24*3600;
rel_sec = 8*3600;      % 08:00
epsT = 1e-9;

day  = floor(t/SEC_PER_DAY);
tod  = mod(t, SEC_PER_DAY);

next_day = day;

while true
    ndow  = mod(next_day,7);
    nweek = floor(next_day/7);

    if ndow == 5 || ndow == 6
        next_day = next_day + 1;
        continue;
    end

    if (nweek == 0) && (ndow == 0)
        next_day = next_day + 1;
        continue;
    end

    if next_day == day
        if tod < rel_sec - epsT
            break;
        else
            next_day = next_day + 1;
            continue;
        end
    else
        break;
    end
end

next_release = next_day*SEC_PER_DAY + rel_sec;
dt = max(next_release - t, 1e-6);

end

== matlab function Design_5new_4weeks_Q3/MATLAB Function 2 ==
  data: t input; cap output




function cap = operator_capacity_p1(t)
%#codegen

SEC_PER_DAY = 24*3600;

day = floor(t/SEC_PER_DAY);     % Day index
tod = mod(t, SEC_PER_DAY);      % Time of day (seconds)
dow = mod(day,7);               % Day of week (0=Mon,...,6=Sun)
week = floor(day/7);            % Week index

% --- Weekend: no operator ---
if dow >= 5
    cap = 0;
    return;
end

% --- Special case: First Monday (week 0) ---
if (week == 0) && (dow == 0)
    % Only 12:00–16:00
    if tod >= 12*3600 && tod < 16*3600
        cap = 1;
    else
        cap = 0;
    end
else
    % Normal weekdays: 08:00–16:00
    if tod >= 8*3600 && tod < 16*3600
        cap = 1;
    else
        cap = 0;
    end
end

end

== matlab function Design_5new_4weeks_Q3/Manual Cleaning/MATLAB Function ==
  data: d input; payload output double size=1


%function payload = fcn(d)
%#codegen

%payload = double(d);

%end

%%

%function payload = fcn(d)
%#codegen

%payload = 2.0;
%payload = uint8(2);
%payload = uint8('2');

%payload = uint8(50);   % ASCII '2'
%payload = '2';

%end

%%

function payload = fcn(d)
%#codegen

if d > 0
    payload = 2.0;   % Manual Cleaning completed
else
    payload = 0.0;
end

end

== matlab function Design_5new_4weeks_Q3/MATLAB Function ==
  data: d input; payload output double size=1


%function payload = fcn(d)
%#codegen

%payload = double(d);

%end


%function payload = fcn(d)
%#codegen

%payload = 1.0;
%payload = uint8(1);
%payload = uint8('1');
%payload = uint8(49);   % ASCII '1'
%payload = '1';

%end

%%

function payload = fcn(d)
%#codegen

if d > 0
    payload = 1.0;   % Blasting completed
else
    payload = 0.0;
end

end

== matlab function Design_5new_4weeks_Q3/MATLAB Function1 ==
  data: d input; payload output double size=1



%function payload = fcn(d)
%#codegen

%payload = double(d);

%end

%%

%function payload = fcn(d)

%#codegen

%payload = 3.0;
%payload = uint8(3);
%payload = uint8('3');
%payload = uint8(51);   % ASCII '3'
%payload = '3';

%end


%%

function payload = fcn(d)
%#codegen

if d > 0
    payload = 3.0;   % Surfacing completed
else
    payload = 0.0;
end

end
